simulink model "RBFNN_IntegralSMC_Simulation"  (R2020b)
settings: Solver=FixedStepAuto  StartTime=0.0  StopTime=60  FixedStep=1e-3  RelTol=1e-3
settings Model: Creator=hellb  LastModifiedBy=Ivan Lopez
settings SolverCC: AlgebraicLoopSolver=LineSearch
settings DataIOCC: ReturnWorkspaceOutputs=off
settings DebuggingCC: ArithmeticOperatorsInVariantConditions=warning
settings SFSimCC: SimUseLocalCustomCode=off  CustomCodeUndefinedFunction=UseInterfaceOnly
settings RTWCC: RTWUseLocalCustomCode=off

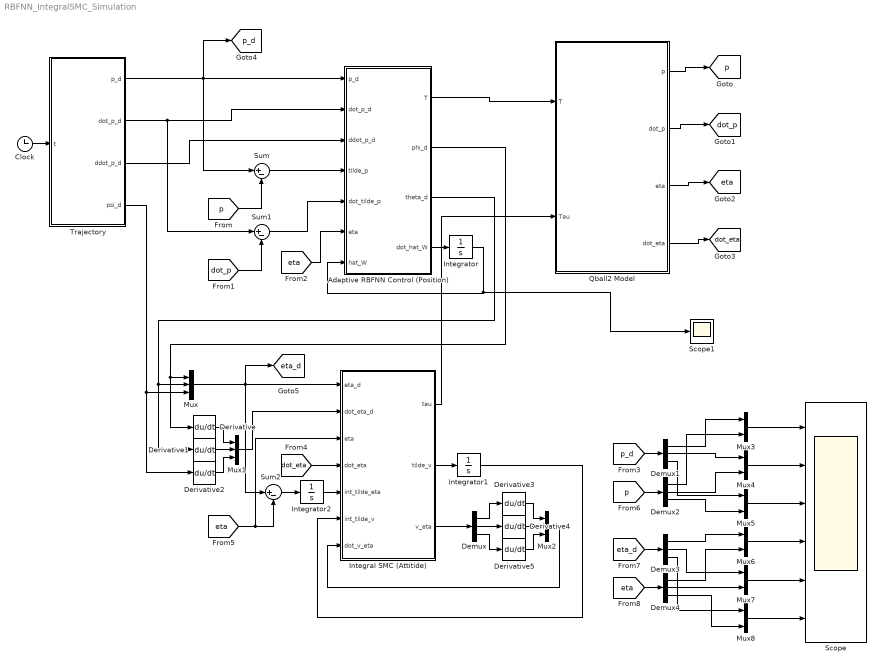
== system RBFNN_IntegralSMC_Simulation ==
  Adaptive RBFNN Control (Position) : MATLAB Function  TreatAsAtomicUnit=on
  Clock : Clock
  Demux{,1..4} (5 alike) : Demux  Outputs=3
  Derivative{,1..5} (6 alike) : Derivative
  Integral SMC (Attitide) : MATLAB Function  TreatAsAtomicUnit=on
  Integrator : Integrator  InitialCondition=0.005*ones(7,3)
  Integrator1 : Integrator  InitialCondition=[0;0;0]
  Integrator2 : Integrator  InitialCondition=[0;0;0]
  Mux : Mux  Inputs=3
  Mux1 : Mux  Inputs=3
  Mux2 : Mux  Inputs=3
  Mux{3..8} (6 alike) : Mux  Inputs=2
  Qball2 Model : Subsystem
  Scope : Scope  NumInputPorts=6
  Scope1 : Scope
  Sum : Sum  Inputs=|+-
  Sum1 : Sum  Inputs=|+-
  Sum2 : Sum  Inputs=|+-
  Trajectory : MATLAB Function  TreatAsAtomicUnit=on
  tag scope: dot_eta=global, dot_p=global, eta=global, eta_d=global, p=global, p_d=global
  wires:
  Adaptive RBFNN Control (Position)/1(T) -> Qball2 Model/1(T)
  [p] -> Sum/2
  Sum/1 -> Adaptive RBFNN Control (Position)/4(tilde_p)
  [dot_p] -> Sum1/2
  Sum1/1 -> Adaptive RBFNN Control (Position)/5(dot_tilde_p)
  Trajectory/1(p_d) -> [p_d], Sum/1, Adaptive RBFNN Control (Position)/1(p_d)
  Trajectory/2(dot_p_d) -> Sum1/1, Adaptive RBFNN Control (Position)/2(dot_p_d)
  Clock/1 -> Trajectory/1(t)
  Trajectory/3(ddot_p_d) -> Adaptive RBFNN Control (Position)/3(ddot_p_d)
  Adaptive RBFNN Control (Position)/4(dot_hat_W) -> Integrator/1
  Integrator/1 -> Scope1/1, Adaptive RBFNN Control (Position)/7(hat_W)
  Qball2 Model/1(p) -> [p]
  Qball2 Model/2(dot_p) -> [dot_p]
  Qball2 Model/3(eta) -> [eta]
  Qball2 Model/4(dot_eta) -> [dot_eta]
  [eta] -> Adaptive RBFNN Control (Position)/6(eta)
  [dot_eta] -> Integral SMC (Attitide)/4(dot_eta)
  Adaptive RBFNN Control (Position)/3(theta_d) -> Derivative1/1, Mux/2
  Adaptive RBFNN Control (Position)/2(phi_d) -> Derivative/1, Mux/1
  Trajectory/4(psi_d) -> Derivative2/1, Mux/3
  Mux/1 -> [eta_d], Sum2/1, Integral SMC (Attitide)/1(eta_d)
  Derivative1/1 -> Mux1/2
  Derivative/1 -> Mux1/1
  Derivative2/1 -> Mux1/3
  Mux1/1 -> Integral SMC (Attitide)/2(dot_eta_d)
  Integral SMC (Attitide)/1(tau) -> Qball2 Model/2(Tau)
  Integral SMC (Attitide)/2(tilde_v) -> Integrator1/1
  Derivative5/1 -> Mux2/3
  Derivative3/1 -> Mux2/1
  Derivative4/1 -> Mux2/2
  Demux/1 -> Derivative3/1
  Demux/2 -> Derivative4/1
  Demux/3 -> Derivative5/1
  Integral SMC (Attitide)/3(v_eta) -> Demux/1
  Mux2/1 -> Integral SMC (Attitide)/7(dot_v_eta)
  Integrator1/1 -> Integral SMC (Attitide)/6(int_tilde_v)
  Integrator2/1 -> Integral SMC (Attitide)/5(int_tilde_eta)
  Sum2/1 -> Integrator2/1
  [eta] -> Integral SMC (Attitide)/3(eta), Sum2/2
  Mux3/1 -> Scope/1
  [p_d] -> Demux1/1
  [p] -> Demux2/1
  [eta] -> Demux4/1
  [eta_d] -> Demux3/1
  Mux4/1 -> Scope/2
  Mux6/1 -> Scope/4
  Mux5/1 -> Scope/3
  Mux7/1 -> Scope/5
  Mux8/1 -> Scope/6
  Demux1/1 -> Mux3/1
  Demux2/1 -> Mux3/2
  Demux1/2 -> Mux4/1
  Demux2/2 -> Mux4/2
  Demux1/3 -> Mux5/1
  Demux2/3 -> Mux5/2
  Demux3/1 -> Mux6/1
  Demux4/1 -> Mux6/2
  Demux3/2 -> Mux7/1
  Demux4/2 -> Mux7/2
  Demux3/3 -> Mux8/1
  Demux4/3 -> Mux8/2

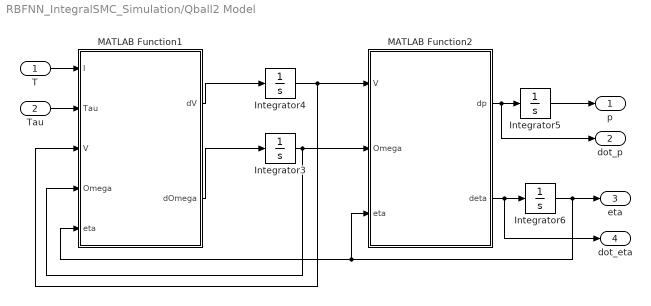
== system RBFNN_IntegralSMC_Simulation/Qball2 Model ==
  T : Inport
  Tau : Inport  Port=2
  Integrator3 : Integrator  InitialCondition=[0;0;0]
  Integrator4 : Integrator  InitialCondition=[0;0;0]
  Integrator5 : Integrator  InitialCondition=[0;0;0.3]  LimitOutput=on  UpperSaturationLimit=[inf;inf;inf]  LowerSaturationLimit=[-inf;-inf;0.3]
  Integrator6 : Integrator  InitialCondition=[0;0;0]
  MATLAB Function1 : MATLAB Function  TreatAsAtomicUnit=on
  MATLAB Function2 : MATLAB Function  TreatAsAtomicUnit=on
  p : Outport  VectorParamsAs1DForOutWhenUnconnected=off
  dot_p : Outport  Port=2  VectorParamsAs1DForOutWhenUnconnected=off
  eta : Outport  Port=3  VectorParamsAs1DForOutWhenUnconnected=off
  dot_eta : Outport  Port=4  VectorParamsAs1DForOutWhenUnconnected=off
  wires:
  MATLAB Function2/2(deta) -> Integrator6/1, dot_eta/1
  MATLAB Function2/1(dp) -> dot_p/1, Integrator5/1
  MATLAB Function1/1(dV) -> Integrator4/1
  MATLAB Function1/2(dOmega) -> Integrator3/1
  Tau/1 -> MATLAB Function1/2(Tau)
  T/1 -> MATLAB Function1/1(I)
  Integrator6/1 -> eta/1, MATLAB Function2/3(eta), MATLAB Function1/5(eta)
  Integrator5/1 -> p/1
  Integrator3/1 -> MATLAB Function1/4(Omega), MATLAB Function2/2(Omega)
  Integrator4/1 -> MATLAB Function1/3(V), MATLAB Function2/1(V)

== matlab function RBFNN_IntegralSMC_Simulation/Trajectory ==
  data: t input; p_d output; dot_p_d output; ddot_p_d output; psi_d output
function [p_d,dot_p_d,ddot_p_d,psi_d] = fcn(t)

x_amp = 0.5;
y_amp = 1;
% z_amp = 0;

x_frec = 2*pi/4;
y_frec = 2*pi/8;
% z_frec = 0;

z_b = 1;

p_d = [x_amp*sin(x_frec*t);
       y_amp*cos(y_frec*t);
       z_b];
   
dot_p_d = [x_frec*x_amp*cos(x_frec*t);
           y_frec*y_amp*-sin(y_frec*t);
           0];
       
ddot_p_d = [x_frec^2*x_amp*-sin(x_frec*t);
            y_frec^2*y_amp*-cos(y_frec*t);
            0];
        
psi_d = 0;

== matlab function RBFNN_IntegralSMC_Simulation/Adaptive RBFNN Control (Position) ==
  data: T output; p_d input; dot_p_d input; ddot_p_d input; tilde_p input; phi_d output; theta_d output; dot_hat_W output; dot_tilde_p input; eta input; hat_W input
function [T, phi_d,theta_d,dot_hat_W] = fcn(p_d, dot_p_d, ddot_p_d, tilde_p, dot_tilde_p, eta, hat_W)
m = 1.79;
g = 9.81;
%% RBFNN parameters
c      = [-1.5,-1,-0.5,0,0.5,1,1.5];
J      = length(c);
sigma  = 5*ones(J,1);
Lambda = 0.85;
A      = 100;
Kv     = 12;
%%
phi   = eta(1);
theta = eta(2);
psi   = eta(3);

M  = diag([1/m 1/m cos(phi)*cos(theta)/m]);
e3 = [0;0;1];

Xin = [tilde_p' dot_tilde_p' p_d' dot_p_d' ddot_p_d'];
P = zeros(J,1);
for i=1:J
    P(i) = exp(-(norm(Xin - c(i))^2)/sigma(i)^2);
end

gamma = dot_tilde_p + Lambda*tilde_p;

dot_hat_W = A*P*gamma';
hat_f = hat_W'*P;
u = M\(g*e3 + hat_f + Kv*gamma);

u1 = u(1)/u(3);
u2 = u(2)/u(3);

T = u(3);

phi_d   = asin(u1*sin(psi) - u2*cos(psi));
theta_d = asin((u1*cos(psi) + u2*sin(psi))/cos(phi_d));

== matlab function RBFNN_IntegralSMC_Simulation/Integral SMC (Attitide) ==
  data: eta_d input; dot_eta_d input; tau output; eta input; dot_eta input; int_tilde_eta input; int_tilde_v input; dot_v_eta input; tilde_v output; v_eta output
function [tau, tilde_v, v_eta]  = fcn(eta_d, dot_eta_d, eta, dot_eta, int_tilde_eta, int_tilde_v, dot_v_eta)

Ixx = 0.03;
Iyy = Ixx;
Izz = 0.04;

kw    = 100;
kn    = 20;
rho_w = 0.001;
rho_n = 0.001;

phi   = eta(1);
theta = eta(2);

dot_phi   = dot_eta(1);
dot_theta = dot_eta(2);
dot_psi   = dot_eta(3);

M_eta = [Ixx 0 -Ixx*sin(theta);
         0 Iyy*cos(phi)^2+Izz*sin(phi)^2 (Iyy-Izz)*cos(phi)*sin(phi)*cos(theta);
         -Ixx*sin(theta) (Iyy-Izz)*cos(phi)*sin(phi)*cos(theta) Ixx*sin(theta)^2+Iyy*sin(phi)^2*cos(theta)^2+Izz*cos(phi)^2*cos(theta)^2];

C12 = (Iyy-Izz)*(dot_theta*cos(phi)*sin(phi)+dot_psi*sin(phi)^2*cos(theta))...
    + (Izz-Iyy)*dot_psi*cos(phi)^2*cos(theta)...
    - Ixx*dot_psi*cos(theta);

C13 = (Izz-Iyy)*dot_psi*cos(phi)*sin(phi)*cos(theta)^2;

C21 = (Izz-Iyy)*(dot_theta*cos(phi)*sin(phi)+dot_psi*sin(phi)^2*cos(theta))...
    + (Iyy-Izz)*dot_psi*cos(phi)^2*cos(theta)...
    + Ixx*dot_psi*cos(theta);

C22 = (Izz-Iyy)*dot_phi*cos(phi)*sin(phi);

C23 = -Ixx*dot_psi*sin(theta)*cos(theta)...
    + Iyy*dot_psi*sin(phi)^2*cos(theta)*sin(theta)...
    + Izz*dot_psi*cos(phi)^2*sin(theta)*cos(theta);

C31 = (Iyy-Izz)*dot_psi*cos(theta)^2*sin(phi)*cos(phi)...
    - Ixx*dot_theta*cos(theta);

C32 = (Izz-Iyy)*(dot_theta*cos(phi)*sin(phi)*sin(theta))...
    + (Iyy-Izz)*dot_phi*cos(phi)^2*cos(theta)...
    + Ixx*dot_psi*sin(theta)*cos(theta)...
    - Iyy*dot_psi*sin(phi)^2*sin(theta)*cos(theta)...
    - Izz*dot_theta*cos(phi)^2*sin(theta)*cos(theta);

C33 = (Iyy-Izz)*dot_phi*cos(phi)*sin(phi)*cos(theta)^2 ...
    - Iyy*dot_theta*sin(phi)^2*cos(theta)*sin(theta)...
    - Izz*dot_theta*cos(phi)^2*cos(theta)*sin(theta)...
    + Ixx*dot_theta*cos(theta)*sin(theta);

C_eta = [0   C12 C13;
         C21 C22 C23;
         C31 C32 C33];
     
tilde_eta = eta_d - eta;

s_w = tilde_eta + kw*int_tilde_eta;

v_eta = dot_eta_d + kw*tilde_eta + rho_w*sign(s_w);

tilde_v = v_eta - dot_eta;
     
s_n = tilde_v + kn*int_tilde_v;
     
tau = M_eta*dot_v_eta + C_eta*dot_eta + rho_n*sign(s_n) + kn*M_eta*tilde_v;

== matlab function RBFNN_IntegralSMC_Simulation/Qball2 Model/MATLAB Function1 ==
  data: I input; Tau input; V input; dV output; Omega input; eta input; dOmega output
function [dV,dOmega] = fcn(I,Tau,V,Omega,eta)

%  TTA = [1.7613 %Parametros identificados 1
%     0.0128
%     0.0151
%     0.0024];

%  TTA = [1.7874 %Parametros identificados 2
%     0.0156
%     0.0186
%     0.0010];

%  TTA = [1.7917 %Parametros identificados 3
%     0.0140
%     0.0148
%     0.0013];

 TTA = [1.79 %Parametros fabricante
    0.03
    0.03
    0.04];

TAUphi = Tau(1);
TAUtta = Tau(2);
TAUpsi = Tau(3);

u = V(1);
v = V(2);
w = V(3);

p = Omega(1);
q = Omega(2);
r = Omega(3);

phi = eta(1);
tta = eta(2);

gbx = -9.8*sin(tta);
gby = 9.8*cos(tta)*sin(phi);
gbz = 9.8*cos(tta)*cos(phi);

  m = TTA(1,1);
Ixx = TTA(2,1);
Iyy = TTA(3,1);
Izz = TTA(4,1);

du = r*v - q*w - gbx;
dv = p*w - r*u - gby;
dw = q*u - p*v - gbz + I/m;
dp = ((Iyy-Izz)*q*r + TAUphi)/Ixx;
dq = ((Izz-Ixx)*p*r + TAUtta)/Iyy;
dr = ((Ixx-Iyy)*p*q + TAUpsi)/Izz;

    dV = [du;dv;dw];
dOmega = [dp;dq;dr];

== matlab function RBFNN_IntegralSMC_Simulation/Qball2 Model/MATLAB Function2 ==
  data: V input; dp output; Omega input; eta input; deta output
function [dp,deta] = fcn(V,Omega,eta)

phi = eta(1);
tta = eta(2);
psi = eta(3);

R = [cos(psi)*cos(tta)  -sin(psi)*cos(phi)+cos(psi)*sin(tta)*sin(phi)   sin(psi)*sin(phi)+cos(psi)*cos(phi)*sin(tta)
     sin(psi)*cos(tta)   cos(psi)*cos(phi)+sin(phi)*sin(tta)*sin(psi)   sin(tta)*sin(psi)*cos(phi)-cos(psi)*sin(phi)
     -sin(tta)           cos(tta)*sin(phi)                              cos(tta)*cos(phi)];
 
W = [1  sin(phi)*tan(tta)   cos(phi)*tan(tta)
     0  cos(phi)           -sin(phi)
     0  sin(phi)/cos(tta)   cos(phi)/cos(tta)];

dp = R*V;
deta = W*Omega;
